simulink model "ParameterBasedTraj"  (R2015a)
settings: Solver=ode45  StartTime=0.0  StopTime=10.0  RelTol=1e-3
undefined symbols (not defined in the file or in its folder): a
libraries: etargetslib x1, dspnetwork x1
settings Model: Creator=marinho  LastModifiedBy=marinho

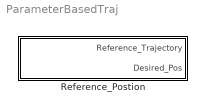
== system ParameterBasedTraj ==
  Reference_Postion : Subsystem

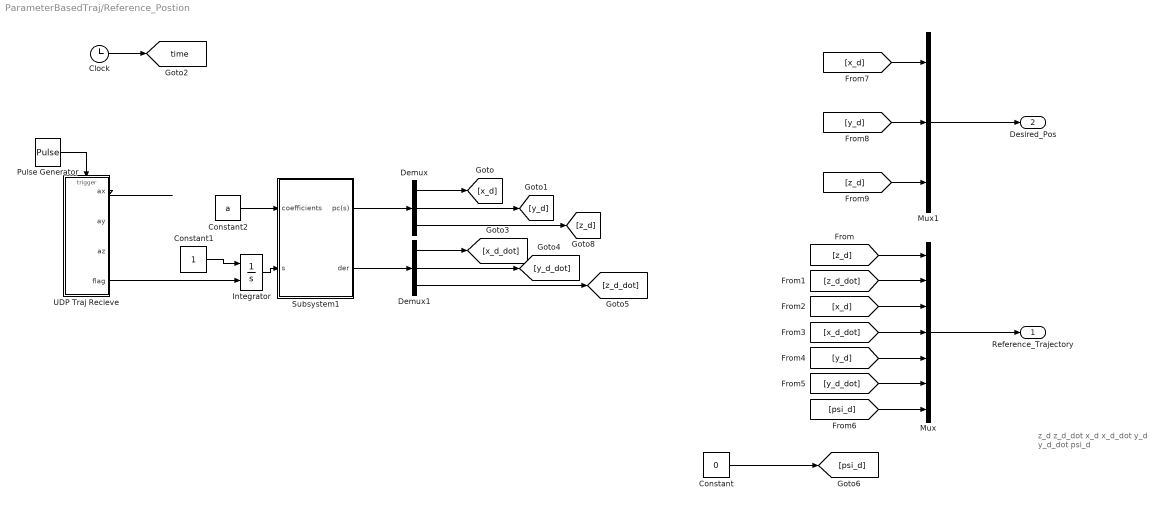
== system ParameterBasedTraj/Reference_Postion ==
  note: z_d
      | z_d_dot
      |
      | x_d
      | x_d_dot
      |
      | y_d
      | y_d_dot
      |
      | psi_d
  Clock : Clock
  Constant : Constant  Value=0
  Constant1 : Constant
  Constant2 : Constant  Value=a
  Demux : Demux  Outputs=3
  Demux1 : Demux  Outputs=3
  Integrator : Integrator  ExternalReset=either
  Mux : Mux  Inputs=7
  Mux1 : Mux  Inputs=3
  Pulse Generator : DiscretePulseGenerator  PulseType=Time based  Period=1/10  PulseWidth=50
  Subsystem1 : Subsystem
  UDP Traj Recieve : Subsystem
  Reference_Trajectory : Outport
  Desired_Pos : Outport  Port=2
  tag scope: time=global
  wires:
  Mux/1 -> Reference_Trajectory/1
  [z_d] -> Mux/1
  [z_d_dot] -> Mux/2
  [x_d] -> Mux/3
  [x_d_dot] -> Mux/4
  [y_d] -> Mux/5
  [y_d_dot] -> Mux/6
  [psi_d] -> Mux/7
  [x_d] -> Mux1/1
  [y_d] -> Mux1/2
  [z_d] -> Mux1/3
  Mux1/1 -> Desired_Pos/1
  Clock/1 -> [time]
  Pulse Generator/1 -> UDP Traj Recieve/Trigger
  Demux1/1 -> [x_d_dot]
  UDP Traj Recieve/1(ax) -> ?
  Constant1/1 -> Integrator/1
  Demux1/2 -> [y_d_dot]
  Constant/1 -> [psi_d]
  Subsystem1/1(pc(s)) -> Demux/1
  Demux/1 -> [x_d]
  Demux/2 -> [y_d]
  Demux/3 -> [z_d]
  Subsystem1/2(der) -> Demux1/1
  Demux1/3 -> [z_d_dot]
  Constant2/1 -> Subsystem1/1(coefficients)
  Integrator/1 -> Subsystem1/2(s)
  UDP Traj Recieve/4(flag) -> Integrator/2

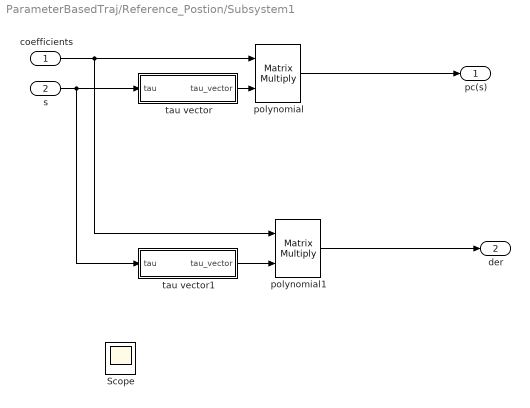
== system ParameterBasedTraj/Reference_Postion/Subsystem1 ==
  coefficients : Inport
  s : Inport  Port=2
  Scope : Scope
  polynomial : Product  Multiplication=Matrix(*)  SaturateOnIntegerOverflow=on  OutDataTypeStr=Inherit: Same as first input
  polynomial1 : Product  Multiplication=Matrix(*)  SaturateOnIntegerOverflow=on  OutDataTypeStr=Inherit: Same as first input
  tau vector : Subsystem
  tau vector1 : Subsystem
  pc(s) : Outport
  der : Outport  Port=2
  wires:
  polynomial/1 -> pc(s)/1
  tau vector/1(tau_vector) -> polynomial/2
  tau vector1/1(tau_vector) -> polynomial1/2
  s/1 -> tau vector1/1(tau), tau vector/1(tau)
  coefficients/1 -> polynomial1/1, polynomial/1
  polynomial1/1 -> der/1

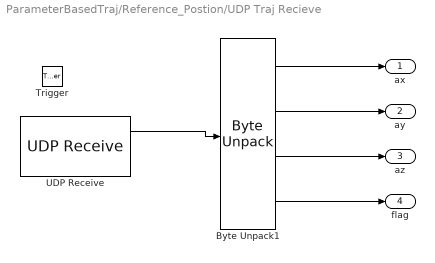
== system ParameterBasedTraj/Reference_Postion/UDP Traj Recieve ==
  Trigger : TriggerPort  PortDimensions=1
  Byte Unpack1 : etargetslib/Byte Unpack  dimensions={8,8,8,1}  datatypes={'double','double','double','double'}  byteAlign=1
  UDP Receive : dspnetwork/UDP Receive  localURL='0.0.0.0'  localPort=25002  remoteURL='127.0.0.1'  remotePort=-1  recvBufferSize=24  dims=24  signalDatatype=uint8  isVarSize=off  showBlockingTime=on  blockingTime=0  sampletime=-1  blockPlatform=HOST
  ax : Outport
  ay : Outport  Port=2
  az : Outport  Port=3
  flag : Outport  Port=4
  wires:
  UDP Receive/1 -> Byte Unpack1/1
  Byte Unpack1/1 -> ax/1
  Byte Unpack1/2 -> ay/1
  Byte Unpack1/3 -> az/1
  Byte Unpack1/4 -> flag/1

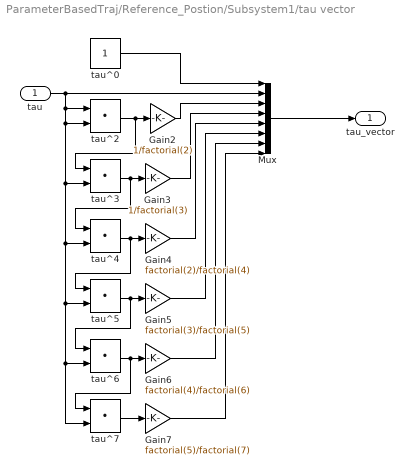
== system ParameterBasedTraj/Reference_Postion/Subsystem1/tau vector ==
  tau : Inport
  Gain2 : Gain  Gain=1/factorial(2)  SaturateOnIntegerOverflow=on  OutDataTypeStr=Inherit: Same as input  ParamDataTypeStr=Inherit: Same as input
  Gain3 : Gain  Gain=1/factorial(3)  SaturateOnIntegerOverflow=on  OutDataTypeStr=Inherit: Same as input  ParamDataTypeStr=Inherit: Same as input
  Gain4 : Gain  Gain=factorial(2)/factorial(4)  SaturateOnIntegerOverflow=on  OutDataTypeStr=Inherit: Same as input  ParamDataTypeStr=Inherit: Same as input
  Gain5 : Gain  Gain=factorial(3)/factorial(5)  SaturateOnIntegerOverflow=on  OutDataTypeStr=Inherit: Same as input  ParamDataTypeStr=Inherit: Same as input
  Gain6 : Gain  Gain=factorial(4)/factorial(6)  SaturateOnIntegerOverflow=on  OutDataTypeStr=Inherit: Same as input  ParamDataTypeStr=Inherit: Same as input
  Gain7 : Gain  Gain=factorial(5)/factorial(7)  SaturateOnIntegerOverflow=on  OutDataTypeStr=Inherit: Same as input  ParamDataTypeStr=Inherit: Same as input
  Mux : Mux  Inputs=8
  tau^0 : Constant
  tau^{2..7} (6 alike) : DotProduct  InputSameDT=on  OutDataTypeStr=Inherit: Inherit via internal rule
  tau_vector : Outport
  wires:
  tau^6/1 -> tau^7/1, Gain6/1
  tau^7/1 -> Gain7/1
  Gain7/1 -> Mux/8
  Gain6/1 -> Mux/7
  Gain4/1 -> Mux/5
  Gain5/1 -> Mux/6
  tau^5/1 -> tau^6/1, Gain5/1
  Gain2/1 -> Mux/3
  Gain3/1 -> Mux/4
  tau^4/1 -> tau^5/1, Gain4/1
  tau^2/1 -> Gain2/1, tau^3/1
  tau^0/1 -> Mux/1
  tau^3/1 -> Gain3/1, tau^4/1
  tau/1 -> tau^7/2, tau^6/2, tau^5/2, tau^4/2, tau^3/2, tau^2/2, tau^2/1, Mux/2
  Mux/1 -> tau_vector/1

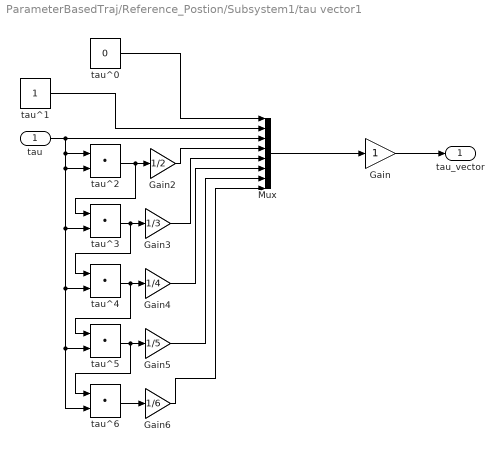
== system ParameterBasedTraj/Reference_Postion/Subsystem1/tau vector1 ==
  tau : Inport
  Gain : Gain
  Gain2 : Gain  Gain=1/2  SaturateOnIntegerOverflow=on  OutDataTypeStr=Inherit: Same as input  ParamDataTypeStr=Inherit: Same as input
  Gain3 : Gain  Gain=1/3  SaturateOnIntegerOverflow=on  OutDataTypeStr=Inherit: Same as input  ParamDataTypeStr=Inherit: Same as input
  Gain4 : Gain  Gain=1/4  SaturateOnIntegerOverflow=on  OutDataTypeStr=Inherit: Same as input  ParamDataTypeStr=Inherit: Same as input
  Gain5 : Gain  Gain=1/5  SaturateOnIntegerOverflow=on  OutDataTypeStr=Inherit: Same as input  ParamDataTypeStr=Inherit: Same as input
  Gain6 : Gain  Gain=1/6  SaturateOnIntegerOverflow=on  OutDataTypeStr=Inherit: Same as input  ParamDataTypeStr=Inherit: Same as input
  Mux : Mux  Inputs=8
  tau^0 : Constant  Value=0
  tau^1 : Constant
  tau^{2..6} (5 alike) : DotProduct  InputSameDT=on  OutDataTypeStr=Inherit: Inherit via internal rule
  tau_vector : Outport
  wires:
  Mux/1 -> Gain/1
  tau^0/1 -> Mux/1
  tau/1 -> Mux/3, tau^2/1, tau^2/2, tau^3/2, tau^4/2, tau^5/2, tau^6/2
  tau^3/1 -> tau^4/1, Gain3/1
  tau^2/1 -> tau^3/1, Gain2/1
  tau^4/1 -> Gain4/1, tau^5/1
  Gain3/1 -> Mux/5
  Gain2/1 -> Mux/4
  tau^5/1 -> Gain5/1, tau^6/1
  Gain5/1 -> Mux/7
  Gain4/1 -> Mux/6
  Gain6/1 -> Mux/8
  tau^6/1 -> Gain6/1
  tau^1/1 -> Mux/2
  Gain/1 -> tau_vector/1
